simulink model "simple_dextair"  (R2018b)
settings: Solver=VariableStepAuto  StartTime=0.0  StopTime=T_simulink  RelTol=1e-3
values from neighbouring files (symbols this model uses):
  a = 1.7*10^(-6)    (= 1.7e-06)    [MAIN.m]
  delta = 0.32    [MAIN.m]
  g = 9.8    [MAIN.m]
  gamma = 3    [MAIN.m]
  k = 22.5    [MAIN.m]
  L = 0.16    [MAIN.m]
  l_0 = 10    [MAIN.m]
  lamda = 12    [MAIN.m]
  m = 2.7    [MAIN.m]
  perturpationAmp = 0    [MAIN.m]
  perturpationFreq = 0    [MAIN.m]
  PID_D_phi = PID_D    (= 19)    [MAIN.m]
  PID_D_psi = PID_D    (= 19)    [MAIN.m]
  PID_D_theta = PID_D    (= 19)    [MAIN.m]
  PID_D_x = PID_D    (= 19)    [MAIN.m]
  PID_D_y = PID_D    (= 19)    [MAIN.m]
  PID_D_z = PID_D    (= 19)    [MAIN.m]
  PID_I_phi = PID_I    (= 2.12)    [MAIN.m]
  PID_I_psi = PID_I    (= 2.12)    [MAIN.m]
  PID_I_theta = PID_I    (= 2.12)    [MAIN.m]
  PID_I_x = PID_I    (= 2.12)    [MAIN.m]
  PID_I_y = PID_I    (= 2.12)    [MAIN.m]
  PID_I_z = PID_I    (= 2.12)    [MAIN.m]
  PID_P_phi = PID_P    (= 12.71)    [MAIN.m]
  PID_P_psi = PID_P    (= 12.71)    [MAIN.m]
  PID_P_theta = PID_P    (= 12.71)    [MAIN.m]
  PID_P_x = PID_P    (= 12.71)    [MAIN.m]
  PID_P_y = PID_P    (= 12.71)    [MAIN.m]
  PID_P_z = PID_P    (= 12.71)    [MAIN.m]
  SMCONTROLTRUE = 0    [MAIN.m]
  to_motor = 0    [MAIN.m]
  W = 0.866    [MAIN.m]
  w_max = 10000000000000    [MAIN.m]
  Z_0 = m*g/k+l_0    (= 11.176)    [MAIN.m]
libraries: simulink x6
settings Model: PacingRate=3  Creator=shaabang  LastModifiedBy=shaabang
settings SolverCC: ZeroCrossControl=DisableAll  ZeroCrossAlgorithm=Adaptive
settings DebuggingCC: IgnoredZcDiagnostic=none

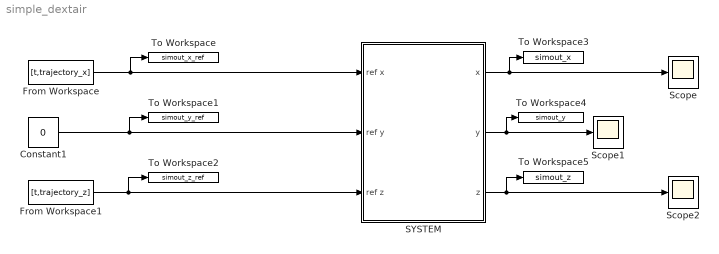
== system simple_dextair ==
  Constant1 : Constant  Value=0
  From Workspace : FromWorkspace  VariableName=[t,trajectory_x]
  From Workspace1 : FromWorkspace  VariableName=[t,trajectory_z]
  SYSTEM : Subsystem
  Scope : Scope
  Scope1 : Scope
  Scope2 : Scope
  To Workspace : ToWorkspace  VariableName=simout_x_ref  SampleTime=-1
  To Workspace1 : ToWorkspace  VariableName=simout_y_ref  SampleTime=-1
  To Workspace2 : ToWorkspace  VariableName=simout_z_ref  SampleTime=-1
  To Workspace3 : ToWorkspace  VariableName=simout_x  SampleTime=-1
  To Workspace4 : ToWorkspace  VariableName=simout_y  SampleTime=-1
  To Workspace5 : ToWorkspace  VariableName=simout_z  SampleTime=-1
  wires:
  SYSTEM/3(z) -> To Workspace5/1, Scope2/1
  SYSTEM/2(y) -> To Workspace4/1, Scope1/1
  SYSTEM/1(x) -> Scope/1, To Workspace3/1
  From Workspace1/1 -> SYSTEM/3(ref z), To Workspace2/1
  From Workspace/1 -> SYSTEM/1(ref x), To Workspace/1
  Constant1/1 -> To Workspace1/1, SYSTEM/2(ref y)

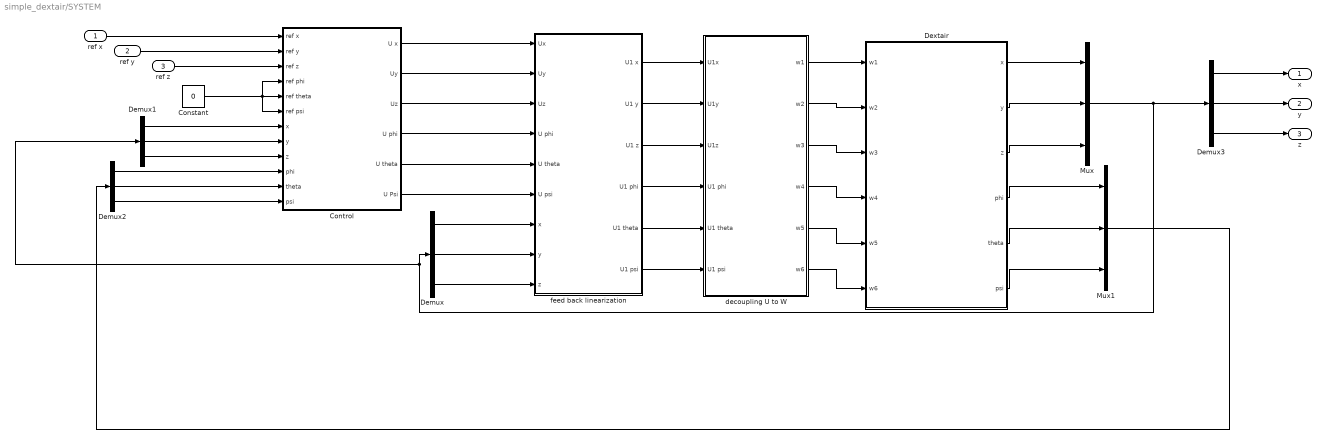
== system simple_dextair/SYSTEM ==
  ref x : Inport
  ref y : Inport  Port=2
  ref z : Inport  Port=3
  Constant : Constant  Value=0
  Control : Subsystem
  Demux{,1..3} (4 alike) : Demux  Outputs=3
  Dextair : Subsystem
  Mux : Mux  Inputs=3
  Mux1 : Mux  Inputs=3
  decoupling U to W : Subsystem
  feed back linearization : Subsystem
  x : Outport
  y : Outport  Port=2
  z : Outport  Port=3
  wires:
  decoupling U to W/5(w5) -> Dextair/5(w5)
  Demux1/2 -> Control/8(y)
  feed back linearization/2(U1 y) -> decoupling U to W/2(U1y)
  ref y/1 -> Control/2(ref y)
  Control/2(Uy) -> feed back linearization/2(Uy)
  feed back linearization/5(U1 theta) -> decoupling U to W/5(U1 theta)
  decoupling U to W/2(w2) -> Dextair/2(w2)
  decoupling U to W/4(w4) -> Dextair/4(w4)
  Dextair/5(theta) -> Mux1/2
  Control/6(U Psi) -> feed back linearization/6(U psi)
  Dextair/1(x) -> Mux/1
  Control/5(U theta) -> feed back linearization/5(U theta)
  Demux2/2 -> Control/11(theta)
  Mux/1 -> Demux3/1, Demux1/1, Demux/1
  decoupling U to W/6(w6) -> Dextair/6(w6)
  feed back linearization/3(U1 z) -> decoupling U to W/3(U1z)
  Demux1/1 -> Control/7(x)
  Demux2/3 -> Control/12(psi)
  decoupling U to W/1(w1) -> Dextair/1(w1)
  Demux/1 -> feed back linearization/7(x)
  Control/4(U phi) -> feed back linearization/4(U phi)
  Control/3(Uz) -> feed back linearization/3(Uz)
  Constant/1 -> Control/6(ref psi), Control/4(ref phi), Control/5(ref theta)
  Demux2/1 -> Control/10(phi)
  Dextair/4(phi) -> Mux1/1
  Demux1/3 -> Control/9(z)
  Dextair/6(psi) -> Mux1/3
  Control/1(U x) -> feed back linearization/1(Ux)
  feed back linearization/6(U1 psi) -> decoupling U to W/6(U1 psi)
  ref x/1 -> Control/1(ref x)
  Dextair/3(z) -> Mux/3
  ref z/1 -> Control/3(ref z)
  Demux3/2 -> y/1
  Demux/2 -> feed back linearization/8(y)
  Demux3/3 -> z/1
  Demux3/1 -> x/1
  Dextair/2(y) -> Mux/2
  feed back linearization/1(U1 x) -> decoupling U to W/1(U1x)
  feed back linearization/4(U1 phi) -> decoupling U to W/4(U1 phi)
  Demux/3 -> feed back linearization/9(z)
  decoupling U to W/3(w3) -> Dextair/3(w3)
  Mux1/1 -> Demux2/1

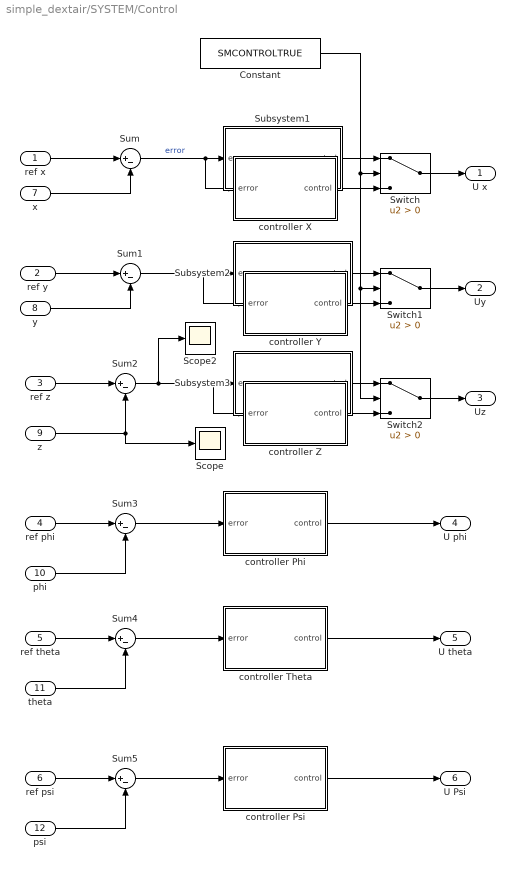
== system simple_dextair/SYSTEM/Control ==
  ref x : Inport
  ref y : Inport  Port=2
  ref z : Inport  Port=3
  ref phi : Inport  Port=4
  ref theta : Inport  Port=5
  ref psi : Inport  Port=6
  x : Inport  Port=7
  y : Inport  Port=8
  z : Inport  Port=9
  phi : Inport  Port=10
  theta : Inport  Port=11
  psi : Inport  Port=12
  Constant : Constant  Value=SMCONTROLTRUE  VectorParams1D=off
  Scope : Scope
  Scope2 : Scope
  Subsystem1 : Subsystem
  Subsystem2 : Subsystem
  Subsystem3 : Subsystem
  Sum{,1..5} (6 alike) : Sum  Inputs=|+-
  Switch : Switch  Criteria=u2 > Threshold
  Switch1 : Switch  Criteria=u2 > Threshold
  Switch2 : Switch  Criteria=u2 > Threshold
  controller Phi : Subsystem
  controller Psi : Subsystem
  controller Theta : Subsystem
  controller X : Subsystem
  controller Y : Subsystem
  controller Z : Subsystem
  U x : Outport
  Uy : Outport  Port=2
  Uz : Outport  Port=3
  U phi : Outport  Port=4
  U theta : Outport  Port=5
  U Psi : Outport  Port=6
  wires:
  controller Psi/1("control ") -> U Psi/1
  controller Theta/1("control ") -> U theta/1
  ref theta/1 -> Sum4/1
  ref y/1 -> Sum1/1
  psi/1 -> Sum5/2
  Sum2/1 -> controller Z/1("error "), Subsystem3/1(error), Scope2/1
  Sum4/1 -> controller Theta/1("error ")
  Sum5/1 -> controller Psi/1("error ")
  Sum1/1 -> controller Y/1("error "), Subsystem2/1(error)
  Sum3/1 -> controller Phi/1("error ")
  x/1 -> Sum/2
  Constant/1 -> Switch2/2, Switch1/2, Switch/2
  Switch2/1 -> Uz/1
  Subsystem1/1(control) -> Switch/1
  theta/1 -> Sum4/2
  Subsystem3/1(control) -> Switch2/1
  ref z/1 -> Sum2/1
  Switch1/1 -> Uy/1
  y/1 -> Sum1/2
  controller Phi/1("control ") -> U phi/1
  ref psi/1 -> Sum5/1
  controller X/1("control ") -> Switch/3
  z/1 -> Scope/1, Sum2/2
  Switch/1 -> U x/1
  phi/1 -> Sum3/2
  Subsystem2/1(control) -> Switch1/1
  ref phi/1 -> Sum3/1
  ref x/1 -> Sum/1
  controller Y/1("control ") -> Switch1/3
  Sum/1 -> controller X/1("error "), Subsystem1/1(error)  "error"
  controller Z/1("control ") -> Switch2/3

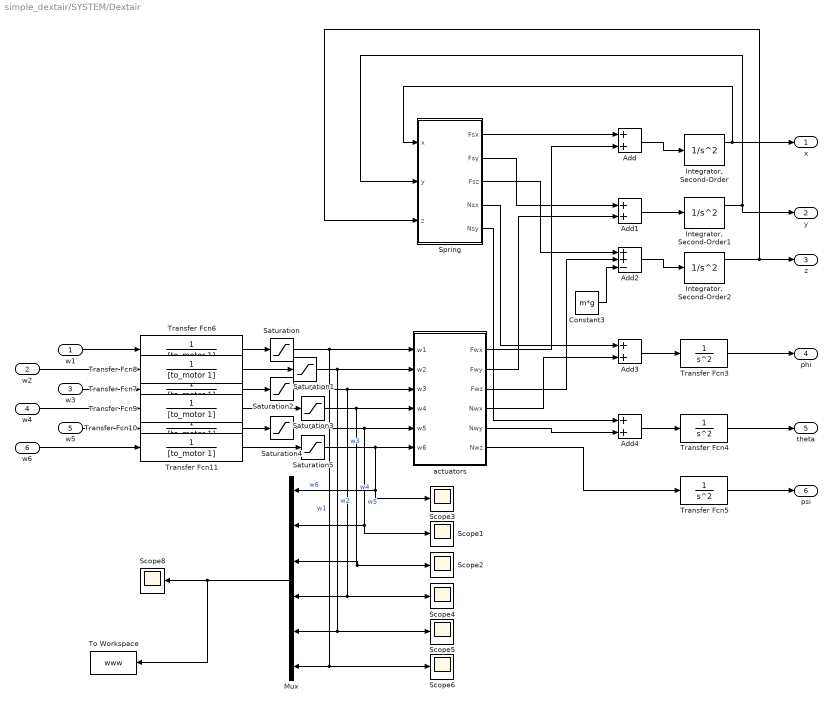
== system simple_dextair/SYSTEM/Dextair ==
  w1 : Inport
  w2 : Inport  Port=2
  w3 : Inport  Port=3
  w4 : Inport  Port=4
  w5 : Inport  Port=5
  w6 : Inport  Port=6
  Add{,1,3..4} (4 alike) : Sum
  Add2 : Sum  Inputs=++-
  Constant3 : Constant  Value=m*g
  "Integrator, Second-Order" : SecondOrderIntegrator  ICX=x0
  "Integrator, Second-Order1" : SecondOrderIntegrator  ICX=y0
  "Integrator, Second-Order2" : SecondOrderIntegrator  ICX=z0
  Mux : Mux  Inputs=6
  Saturation{,1..5} (6 alike) : Saturate  UpperLimit=w_max  LowerLimit=-w_max
  Scope{1..6,8} (7 alike) : Scope
  Spring : Subsystem
  To Workspace : ToWorkspace  VariableName=www  SampleTime=-1
  Transfer Fcn{6..11} (6 alike) : TransferFcn  Denominator=[to_motor 1]
  Transfer Fcn3 : TransferFcn  Denominator=[1 0 0]
  Transfer Fcn4 : TransferFcn  Denominator=[1 0 0]
  Transfer Fcn5 : TransferFcn  Denominator=[1 0 0]
  actuators : Subsystem
  x : Outport
  y : Outport  Port=2
  z : Outport  Port=3
  phi : Outport  Port=4
  theta : Outport  Port=5
  psi : Outport  Port=6
  wires:
  actuators/3(Fwz) -> Add2/2
  Spring/1(Fsx) -> Add/1
  Spring/5(Nsy) -> Add4/1
  Constant3/1 -> Add2/3
  Add3/1 -> Transfer Fcn3/1
  actuators/6(Nwz) -> Transfer Fcn5/1
  Add2/1 -> "Integrator, Second-Order2"/1
  Transfer Fcn5/1 -> psi/1
  Transfer Fcn3/1 -> phi/1
  Transfer Fcn4/1 -> theta/1
  "Integrator, Second-Order1"/1 -> y/1, Spring/2(y)
  Spring/2(Fsy) -> Add1/1
  actuators/1(Fwx) -> Add/2
  "Integrator, Second-Order"/1 -> x/1, Spring/1(x)
  Spring/4(Nsx) -> Add3/1
  Add1/1 -> "Integrator, Second-Order1"/1
  actuators/2(Fwy) -> Add1/2
  Spring/3(Fsz) -> Add2/1
  Add4/1 -> Transfer Fcn4/1
  Add/1 -> "Integrator, Second-Order"/1
  "Integrator, Second-Order2"/1 -> z/1, Spring/3(z)
  actuators/4(Nwx) -> Add3/2
  actuators/5(Nwy) -> Add4/2
  Transfer Fcn9/1 -> Saturation3/1
  Saturation4/1 -> actuators/5(w5), Scope1/1, Mux/2  "w5"
  Transfer Fcn7/1 -> Saturation2/1
  Saturation5/1 -> Scope3/1, Mux/1, actuators/6(w6)  "w6"
  Saturation3/1 -> actuators/4(w4), Scope2/1, Mux/3  "w4"
  Mux/1 -> To Workspace/1, Scope8/1
  Saturation/1 -> actuators/1(w1), Scope6/1, Mux/6  "w1"
  Transfer Fcn10/1 -> Saturation4/1
  Saturation2/1 -> actuators/3(w3), Scope4/1, Mux/4  "w3"
  Saturation1/1 -> actuators/2(w2), Scope5/1, Mux/5  "w2"
  Transfer Fcn8/1 -> Saturation1/1
  Transfer Fcn6/1 -> Saturation/1
  Transfer Fcn11/1 -> Saturation5/1
  w1/1 -> Transfer Fcn6/1
  w2/1 -> Transfer Fcn8/1
  w3/1 -> Transfer Fcn7/1
  w4/1 -> Transfer Fcn9/1
  w5/1 -> Transfer Fcn10/1
  w6/1 -> Transfer Fcn11/1

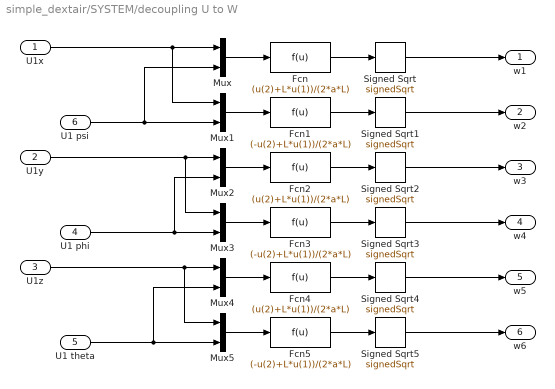
== system simple_dextair/SYSTEM/decoupling U to W ==
  U1x : Inport
  U1y : Inport  Port=2
  U1z : Inport  Port=3
  U1 phi : Inport  Port=4
  U1 theta : Inport  Port=5
  U1 psi : Inport  Port=6
  Fcn : Fcn  Expr=(u(2)+L*u(1))/(2*a*L)
  Fcn1 : Fcn  Expr=(-u(2)+L*u(1))/(2*a*L)
  Fcn2 : Fcn  Expr=(u(2)+L*u(1))/(2*a*L)
  Fcn3 : Fcn  Expr=(-u(2)+L*u(1))/(2*a*L)
  Fcn4 : Fcn  Expr=(u(2)+L*u(1))/(2*a*L)
  Fcn5 : Fcn  Expr=(-u(2)+L*u(1))/(2*a*L)
  Mux{,1..5} (6 alike) : Mux  Inputs=2
  Signed Sqrt{,1..5} (6 alike) : Sqrt  Operator=signedSqrt  SaturateOnIntegerOverflow=on
  w1 : Outport
  w2 : Outport  Port=2
  w3 : Outport  Port=3
  w4 : Outport  Port=4
  w5 : Outport  Port=5
  w6 : Outport  Port=6
  wires:
  Mux2/1 -> Fcn2/1
  Mux1/1 -> Fcn1/1
  Fcn5/1 -> Signed Sqrt5/1
  U1z/1 -> Mux5/1, Mux4/1
  Fcn3/1 -> Signed Sqrt3/1
  U1 theta/1 -> Mux4/2, Mux5/2
  Signed Sqrt2/1 -> w3/1
  Fcn/1 -> Signed Sqrt/1
  Mux3/1 -> Fcn3/1
  U1 psi/1 -> Mux/2, Mux1/2
  Fcn2/1 -> Signed Sqrt2/1
  Signed Sqrt4/1 -> w5/1
  Signed Sqrt5/1 -> w6/1
  Fcn1/1 -> Signed Sqrt1/1
  Signed Sqrt3/1 -> w4/1
  Signed Sqrt1/1 -> w2/1
  Mux/1 -> Fcn/1
  U1 phi/1 -> Mux2/2, Mux3/2
  U1x/1 -> Mux1/1, Mux/1
  U1y/1 -> Mux3/1, Mux2/1
  Mux5/1 -> Fcn5/1
  Fcn4/1 -> Signed Sqrt4/1
  Signed Sqrt/1 -> w1/1
  Mux4/1 -> Fcn4/1

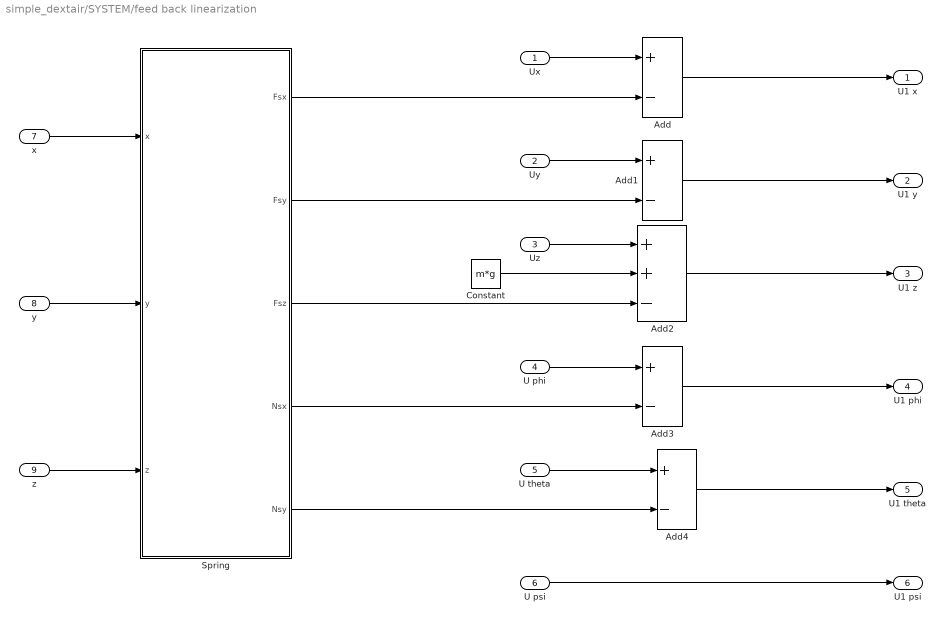
== system simple_dextair/SYSTEM/feed back linearization ==
  Ux : Inport
  Uy : Inport  Port=2
  Uz : Inport  Port=3
  U phi : Inport  Port=4
  U theta : Inport  Port=5
  U psi : Inport  Port=6
  x : Inport  Port=7
  y : Inport  Port=8
  z : Inport  Port=9
  Add{,1,3..4} (4 alike) : Sum  Inputs=+-
  Add2 : Sum  Inputs=++-
  Constant : Constant  Value=m*g
  Spring : Subsystem
  U1 x : Outport
  U1 y : Outport  Port=2
  U1 z : Outport  Port=3
  U1 phi : Outport  Port=4
  U1 theta : Outport  Port=5
  U1 psi : Outport  Port=6
  wires:
  U psi/1 -> U1 psi/1
  Add/1 -> U1 x/1
  Spring/4(Nsx) -> Add3/2
  Uy/1 -> Add1/1
  z/1 -> Spring/3(z)
  y/1 -> Spring/2(y)
  Spring/5(Nsy) -> Add4/2
  Constant/1 -> Add2/2
  U phi/1 -> Add3/1
  Add2/1 -> U1 z/1
  Add4/1 -> U1 theta/1
  Spring/1(Fsx) -> Add/2
  U theta/1 -> Add4/1
  x/1 -> Spring/1(x)
  Spring/3(Fsz) -> Add2/3
  Ux/1 -> Add/1
  Add1/1 -> U1 y/1
  Add3/1 -> U1 phi/1
  Uz/1 -> Add2/1
  Spring/2(Fsy) -> Add1/2

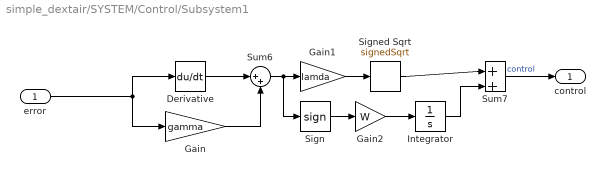
== system simple_dextair/SYSTEM/Control/Subsystem1 ==
  error : Inport
  Derivative : Derivative
  Gain : Gain  Gain=gamma
  Gain1 : Gain  Gain=lamda
  Gain2 : Gain  Gain=W
  Integrator : Integrator
  Sign : Signum
  Signed Sqrt : Sqrt  Operator=signedSqrt  SaturateOnIntegerOverflow=on
  Sum6 : Sum  Inputs=|++
  Sum7 : Sum  Inputs=|++
  control : Outport
  wires:
  Sum7/1 -> control/1  "control"
  Sign/1 -> Gain2/1
  error/1 -> Derivative/1, Gain/1
  Derivative/1 -> Sum6/1
  Gain2/1 -> Integrator/1
  Signed Sqrt/1 -> Sum7/1
  Gain/1 -> Sum6/2
  Gain1/1 -> Signed Sqrt/1
  Sum6/1 -> Gain1/1, Sign/1
  Integrator/1 -> Sum7/2

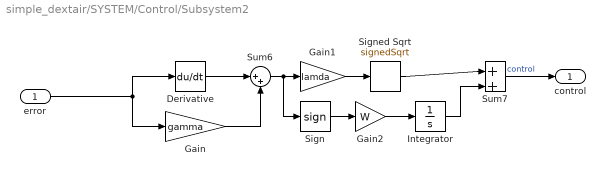
== system simple_dextair/SYSTEM/Control/Subsystem2 ==
  error : Inport
  Derivative : Derivative
  Gain : Gain  Gain=gamma
  Gain1 : Gain  Gain=lamda
  Gain2 : Gain  Gain=W
  Integrator : Integrator
  Sign : Signum
  Signed Sqrt : Sqrt  Operator=signedSqrt  SaturateOnIntegerOverflow=on
  Sum6 : Sum  Inputs=|++
  Sum7 : Sum  Inputs=|++
  control : Outport
  wires:
  Integrator/1 -> Sum7/2
  Sum6/1 -> Sign/1, Gain1/1
  Gain1/1 -> Signed Sqrt/1
  Gain/1 -> Sum6/2
  Signed Sqrt/1 -> Sum7/1
  Gain2/1 -> Integrator/1
  Derivative/1 -> Sum6/1
  error/1 -> Gain/1, Derivative/1
  Sign/1 -> Gain2/1
  Sum7/1 -> control/1  "control"

== system simple_dextair/SYSTEM/Control/Subsystem3 ==
  error : Inport
  Derivative : Derivative
  Gain : Gain  Gain=gamma
  Gain1 : Gain  Gain=lamda
  Gain2 : Gain  Gain=W
  Integrator : Integrator
  Sign : Signum
  Signed Sqrt : Sqrt  Operator=signedSqrt  SaturateOnIntegerOverflow=on
  Sum6 : Sum  Inputs=|++
  Sum7 : Sum  Inputs=|++
  control : Outport
  wires:
  Sum7/1 -> control/1  "control"
  Sign/1 -> Gain2/1
  error/1 -> Derivative/1, Gain/1
  Derivative/1 -> Sum6/1
  Gain2/1 -> Integrator/1
  Signed Sqrt/1 -> Sum7/1
  Gain/1 -> Sum6/2
  Gain1/1 -> Signed Sqrt/1
  Sum6/1 -> Gain1/1, Sign/1
  Integrator/1 -> Sum7/2

== system simple_dextair/SYSTEM/Control/controller Phi ==
  "error " : Inport
  PID Controller : simulink/Continuous/PID Controller  Controller=PID  Form=Parallel  TimeDomain=Continuous-time  SampleTime=-1  IntegratorMethod=Forward Euler  FilterMethod=Forward Euler  ControllerParametersSource=internal  P=PID_P_phi  I=PID_I_phi  D=PID_D_phi  UseFilter=on  N=100  TunerSelectOption=Transfer Function Based (PID Tuner App)  InitialConditionSource=internal  InitialConditionForIntegrator=0  InitialConditionForFilter=0  DifferentiatorICPrevScaledInput=0  ExternalReset=none  TrackingMode=off  Kt=1  LimitOutput=off  UpperSaturationLimit=inf  LowerSaturationLimit=-inf  LinearizeAsGain=on  AntiWindupMode=none  Kb=1  POutMin=[]  POutMax=[]  IOutMin=[]  IOutMax=[]  DOutMin=[]  DOutMax=[]  NOutMin=[]  NOutMax=[]  SumOutMin=[]  SumOutMax=[]  SaturationOutMin=[]  SaturationOutMax=[]  PParamMin=[]  PParamMax=[]  IParamMin=[]  IParamMax=[]  DParamMin=[]  DParamMax=[]  NParamMin=[]  NParamMax=[]  KbParamMin=[]  KbParamMax=[]  KtParamMin=[]  KtParamMax=[]  KbOutMin=[]  KbOutMax=[]  KtOutMin=[]  KtOutMax=[]  IntegratorOutMin=[]  IntegratorOutMax=[]  FilterOutMin=[]  FilterOutMax=[]  SumI1OutMin=[]  SumI1OutMax=[]  SumI2OutMin=[]  SumI2OutMax=[]  SumI3OutMin=[]  SumI3OutMax=[]  SumI4OutMin=[]  SumI4OutMax=[]  SumDOutMin=[]  SumDOutMax=[]  DifferentiatorOutMin=[]  DifferentiatorOutMax=[]  FilterDiffOutCoefMin=[]  FilterDiffOutCoefMax=[]  ReciprocalOutMin=[]  ReciprocalOutMax=[]  SumDenOutMin=[]  SumDenOutMax=[]  SumNumOutMin=[]  SumNumOutMax=[]  DivideOutMin=[]  DivideOutMax=[]  IntegratorContinuousStateAttributes=''  IntegratorStateMustResolveToSignalObject=off  IntegratorRTWStateStorageClass=Auto  FilterContinuousStateAttributes=''  FilterStateMustResolveToSignalObject=off  FilterRTWStateStorageClass=Auto  ParallelPVariant=InternalParameters  IdealPVariant=Disabled  IVariant=InternalParameters  DVariant=InternalParameters  IntegratorVariant=Continuous  SatVariant=Disabled  AWVariant=Passthrough  PCopyVariant=Disabled  TRVariant=Disabled  FdbkBlocksVariant=Forward  IdealPFdbkVariant=Disabled  SatFdbkVariant=Disabled  DerivativeFilterVariant=ContFilter  NVariant=InternalParameters  NCopyVariant=Disabled  FilterICVariant=InternalICsFilter  IntegratorICVariant=InternalICs  ExternalResetVariant=Disabled  TRSumVariant=Passthrough  SumFdbkVariant=Disabled  SumVariant=Sum_PID
  "control " : Outport
  wires:
  PID Controller/1 -> "control "/1
  "error "/1 -> PID Controller/1

== system simple_dextair/SYSTEM/Control/controller Psi ==
  "error " : Inport
  PID Controller : simulink/Continuous/PID Controller  Controller=PID  Form=Parallel  TimeDomain=Continuous-time  SampleTime=-1  IntegratorMethod=Forward Euler  FilterMethod=Forward Euler  ControllerParametersSource=internal  P=PID_P_psi  I=PID_I_psi  D=PID_D_psi  UseFilter=on  N=100  TunerSelectOption=Transfer Function Based (PID Tuner App)  InitialConditionSource=internal  InitialConditionForIntegrator=0  InitialConditionForFilter=0  DifferentiatorICPrevScaledInput=0  ExternalReset=none  TrackingMode=off  Kt=1  LimitOutput=off  UpperSaturationLimit=inf  LowerSaturationLimit=-inf  LinearizeAsGain=on  AntiWindupMode=none  Kb=1  POutMin=[]  POutMax=[]  IOutMin=[]  IOutMax=[]  DOutMin=[]  DOutMax=[]  NOutMin=[]  NOutMax=[]  SumOutMin=[]  SumOutMax=[]  SaturationOutMin=[]  SaturationOutMax=[]  PParamMin=[]  PParamMax=[]  IParamMin=[]  IParamMax=[]  DParamMin=[]  DParamMax=[]  NParamMin=[]  NParamMax=[]  KbParamMin=[]  KbParamMax=[]  KtParamMin=[]  KtParamMax=[]  KbOutMin=[]  KbOutMax=[]  KtOutMin=[]  KtOutMax=[]  IntegratorOutMin=[]  IntegratorOutMax=[]  FilterOutMin=[]  FilterOutMax=[]  SumI1OutMin=[]  SumI1OutMax=[]  SumI2OutMin=[]  SumI2OutMax=[]  SumI3OutMin=[]  SumI3OutMax=[]  SumI4OutMin=[]  SumI4OutMax=[]  SumDOutMin=[]  SumDOutMax=[]  DifferentiatorOutMin=[]  DifferentiatorOutMax=[]  FilterDiffOutCoefMin=[]  FilterDiffOutCoefMax=[]  ReciprocalOutMin=[]  ReciprocalOutMax=[]  SumDenOutMin=[]  SumDenOutMax=[]  SumNumOutMin=[]  SumNumOutMax=[]  DivideOutMin=[]  DivideOutMax=[]  IntegratorContinuousStateAttributes=''  IntegratorStateMustResolveToSignalObject=off  IntegratorRTWStateStorageClass=Auto  FilterContinuousStateAttributes=''  FilterStateMustResolveToSignalObject=off  FilterRTWStateStorageClass=Auto  ParallelPVariant=InternalParameters  IdealPVariant=Disabled  IVariant=InternalParameters  DVariant=InternalParameters  IntegratorVariant=Continuous  SatVariant=Disabled  AWVariant=Passthrough  PCopyVariant=Disabled  TRVariant=Disabled  FdbkBlocksVariant=Forward  IdealPFdbkVariant=Disabled  SatFdbkVariant=Disabled  DerivativeFilterVariant=ContFilter  NVariant=InternalParameters  NCopyVariant=Disabled  FilterICVariant=InternalICsFilter  IntegratorICVariant=InternalICs  ExternalResetVariant=Disabled  TRSumVariant=Passthrough  SumFdbkVariant=Disabled  SumVariant=Sum_PID
  "control " : Outport
  wires:
  PID Controller/1 -> "control "/1
  "error "/1 -> PID Controller/1

== system simple_dextair/SYSTEM/Control/controller Theta ==
  "error " : Inport
  PID Controller : simulink/Continuous/PID Controller  Controller=PID  Form=Parallel  TimeDomain=Continuous-time  SampleTime=-1  IntegratorMethod=Forward Euler  FilterMethod=Forward Euler  ControllerParametersSource=internal  P=PID_P_theta  I=PID_I_theta  D=PID_D_theta  UseFilter=on  N=100  TunerSelectOption=Transfer Function Based (PID Tuner App)  InitialConditionSource=internal  InitialConditionForIntegrator=0  InitialConditionForFilter=0  DifferentiatorICPrevScaledInput=0  ExternalReset=none  TrackingMode=off  Kt=1  LimitOutput=off  UpperSaturationLimit=inf  LowerSaturationLimit=-inf  LinearizeAsGain=on  AntiWindupMode=none  Kb=1  POutMin=[]  POutMax=[]  IOutMin=[]  IOutMax=[]  DOutMin=[]  DOutMax=[]  NOutMin=[]  NOutMax=[]  SumOutMin=[]  SumOutMax=[]  SaturationOutMin=[]  SaturationOutMax=[]  PParamMin=[]  PParamMax=[]  IParamMin=[]  IParamMax=[]  DParamMin=[]  DParamMax=[]  NParamMin=[]  NParamMax=[]  KbParamMin=[]  KbParamMax=[]  KtParamMin=[]  KtParamMax=[]  KbOutMin=[]  KbOutMax=[]  KtOutMin=[]  KtOutMax=[]  IntegratorOutMin=[]  IntegratorOutMax=[]  FilterOutMin=[]  FilterOutMax=[]  SumI1OutMin=[]  SumI1OutMax=[]  SumI2OutMin=[]  SumI2OutMax=[]  SumI3OutMin=[]  SumI3OutMax=[]  SumI4OutMin=[]  SumI4OutMax=[]  SumDOutMin=[]  SumDOutMax=[]  DifferentiatorOutMin=[]  DifferentiatorOutMax=[]  FilterDiffOutCoefMin=[]  FilterDiffOutCoefMax=[]  ReciprocalOutMin=[]  ReciprocalOutMax=[]  SumDenOutMin=[]  SumDenOutMax=[]  SumNumOutMin=[]  SumNumOutMax=[]  DivideOutMin=[]  DivideOutMax=[]  IntegratorContinuousStateAttributes=''  IntegratorStateMustResolveToSignalObject=off  IntegratorRTWStateStorageClass=Auto  FilterContinuousStateAttributes=''  FilterStateMustResolveToSignalObject=off  FilterRTWStateStorageClass=Auto  ParallelPVariant=InternalParameters  IdealPVariant=Disabled  IVariant=InternalParameters  DVariant=InternalParameters  IntegratorVariant=Continuous  SatVariant=Disabled  AWVariant=Passthrough  PCopyVariant=Disabled  TRVariant=Disabled  FdbkBlocksVariant=Forward  IdealPFdbkVariant=Disabled  SatFdbkVariant=Disabled  DerivativeFilterVariant=ContFilter  NVariant=InternalParameters  NCopyVariant=Disabled  FilterICVariant=InternalICsFilter  IntegratorICVariant=InternalICs  ExternalResetVariant=Disabled  TRSumVariant=Passthrough  SumFdbkVariant=Disabled  SumVariant=Sum_PID
  "control " : Outport
  wires:
  PID Controller/1 -> "control "/1
  "error "/1 -> PID Controller/1

== system simple_dextair/SYSTEM/Control/controller X ==
  "error " : Inport
  PID Controller : simulink/Continuous/PID Controller  Controller=PID  Form=Parallel  TimeDomain=Continuous-time  SampleTime=-1  IntegratorMethod=Forward Euler  FilterMethod=Forward Euler  ControllerParametersSource=internal  P=PID_P_x  I=PID_I_x  D=PID_D_x  UseFilter=on  N=100  TunerSelectOption=Transfer Function Based (PID Tuner App)  InitialConditionSource=internal  InitialConditionForIntegrator=0  InitialConditionForFilter=0  DifferentiatorICPrevScaledInput=0  ExternalReset=none  TrackingMode=off  Kt=1  LimitOutput=off  UpperSaturationLimit=inf  LowerSaturationLimit=-inf  LinearizeAsGain=on  AntiWindupMode=none  Kb=1  POutMin=[]  POutMax=[]  IOutMin=[]  IOutMax=[]  DOutMin=[]  DOutMax=[]  NOutMin=[]  NOutMax=[]  SumOutMin=[]  SumOutMax=[]  SaturationOutMin=[]  SaturationOutMax=[]  PParamMin=[]  PParamMax=[]  IParamMin=[]  IParamMax=[]  DParamMin=[]  DParamMax=[]  NParamMin=[]  NParamMax=[]  KbParamMin=[]  KbParamMax=[]  KtParamMin=[]  KtParamMax=[]  KbOutMin=[]  KbOutMax=[]  KtOutMin=[]  KtOutMax=[]  IntegratorOutMin=[]  IntegratorOutMax=[]  FilterOutMin=[]  FilterOutMax=[]  SumI1OutMin=[]  SumI1OutMax=[]  SumI2OutMin=[]  SumI2OutMax=[]  SumI3OutMin=[]  SumI3OutMax=[]  SumI4OutMin=[]  SumI4OutMax=[]  SumDOutMin=[]  SumDOutMax=[]  DifferentiatorOutMin=[]  DifferentiatorOutMax=[]  FilterDiffOutCoefMin=[]  FilterDiffOutCoefMax=[]  ReciprocalOutMin=[]  ReciprocalOutMax=[]  SumDenOutMin=[]  SumDenOutMax=[]  SumNumOutMin=[]  SumNumOutMax=[]  DivideOutMin=[]  DivideOutMax=[]  IntegratorContinuousStateAttributes=''  IntegratorStateMustResolveToSignalObject=off  IntegratorRTWStateStorageClass=Auto  FilterContinuousStateAttributes=''  FilterStateMustResolveToSignalObject=off  FilterRTWStateStorageClass=Auto  ParallelPVariant=InternalParameters  IdealPVariant=Disabled  IVariant=InternalParameters  DVariant=InternalParameters  IntegratorVariant=Continuous  SatVariant=Disabled  AWVariant=Passthrough  PCopyVariant=Disabled  TRVariant=Disabled  FdbkBlocksVariant=Forward  IdealPFdbkVariant=Disabled  SatFdbkVariant=Disabled  DerivativeFilterVariant=ContFilter  NVariant=InternalParameters  NCopyVariant=Disabled  FilterICVariant=InternalICsFilter  IntegratorICVariant=InternalICs  ExternalResetVariant=Disabled  TRSumVariant=Passthrough  SumFdbkVariant=Disabled  SumVariant=Sum_PID
  "control " : Outport
  wires:
  PID Controller/1 -> "control "/1
  "error "/1 -> PID Controller/1

== system simple_dextair/SYSTEM/Control/controller Y ==
  "error " : Inport
  PID Controller : simulink/Continuous/PID Controller  Controller=PID  Form=Parallel  TimeDomain=Continuous-time  SampleTime=-1  IntegratorMethod=Forward Euler  FilterMethod=Forward Euler  ControllerParametersSource=internal  P=PID_P_y  I=PID_I_y  D=PID_D_y  UseFilter=on  N=100  TunerSelectOption=Transfer Function Based (PID Tuner App)  InitialConditionSource=internal  InitialConditionForIntegrator=0  InitialConditionForFilter=0  DifferentiatorICPrevScaledInput=0  ExternalReset=none  TrackingMode=off  Kt=1  LimitOutput=off  UpperSaturationLimit=inf  LowerSaturationLimit=-inf  LinearizeAsGain=on  AntiWindupMode=none  Kb=1  POutMin=[]  POutMax=[]  IOutMin=[]  IOutMax=[]  DOutMin=[]  DOutMax=[]  NOutMin=[]  NOutMax=[]  SumOutMin=[]  SumOutMax=[]  SaturationOutMin=[]  SaturationOutMax=[]  PParamMin=[]  PParamMax=[]  IParamMin=[]  IParamMax=[]  DParamMin=[]  DParamMax=[]  NParamMin=[]  NParamMax=[]  KbParamMin=[]  KbParamMax=[]  KtParamMin=[]  KtParamMax=[]  KbOutMin=[]  KbOutMax=[]  KtOutMin=[]  KtOutMax=[]  IntegratorOutMin=[]  IntegratorOutMax=[]  FilterOutMin=[]  FilterOutMax=[]  SumI1OutMin=[]  SumI1OutMax=[]  SumI2OutMin=[]  SumI2OutMax=[]  SumI3OutMin=[]  SumI3OutMax=[]  SumI4OutMin=[]  SumI4OutMax=[]  SumDOutMin=[]  SumDOutMax=[]  DifferentiatorOutMin=[]  DifferentiatorOutMax=[]  FilterDiffOutCoefMin=[]  FilterDiffOutCoefMax=[]  ReciprocalOutMin=[]  ReciprocalOutMax=[]  SumDenOutMin=[]  SumDenOutMax=[]  SumNumOutMin=[]  SumNumOutMax=[]  DivideOutMin=[]  DivideOutMax=[]  IntegratorContinuousStateAttributes=''  IntegratorStateMustResolveToSignalObject=off  IntegratorRTWStateStorageClass=Auto  FilterContinuousStateAttributes=''  FilterStateMustResolveToSignalObject=off  FilterRTWStateStorageClass=Auto  ParallelPVariant=InternalParameters  IdealPVariant=Disabled  IVariant=InternalParameters  DVariant=InternalParameters  IntegratorVariant=Continuous  SatVariant=Disabled  AWVariant=Passthrough  PCopyVariant=Disabled  TRVariant=Disabled  FdbkBlocksVariant=Forward  IdealPFdbkVariant=Disabled  SatFdbkVariant=Disabled  DerivativeFilterVariant=ContFilter  NVariant=InternalParameters  NCopyVariant=Disabled  FilterICVariant=InternalICsFilter  IntegratorICVariant=InternalICs  ExternalResetVariant=Disabled  TRSumVariant=Passthrough  SumFdbkVariant=Disabled  SumVariant=Sum_PID
  "control " : Outport
  wires:
  "error "/1 -> PID Controller/1
  PID Controller/1 -> "control "/1

== system simple_dextair/SYSTEM/Control/controller Z ==
  "error " : Inport
  PID Controller : simulink/Continuous/PID Controller  Controller=PID  Form=Parallel  TimeDomain=Continuous-time  SampleTime=-1  IntegratorMethod=Forward Euler  FilterMethod=Forward Euler  ControllerParametersSource=internal  P=PID_P_z  I=PID_I_z  D=PID_D_z  UseFilter=on  N=100  TunerSelectOption=Transfer Function Based (PID Tuner App)  InitialConditionSource=internal  InitialConditionForIntegrator=0  InitialConditionForFilter=0  DifferentiatorICPrevScaledInput=0  ExternalReset=none  TrackingMode=off  Kt=1  LimitOutput=off  UpperSaturationLimit=inf  LowerSaturationLimit=-inf  LinearizeAsGain=on  AntiWindupMode=none  Kb=1  POutMin=[]  POutMax=[]  IOutMin=[]  IOutMax=[]  DOutMin=[]  DOutMax=[]  NOutMin=[]  NOutMax=[]  SumOutMin=[]  SumOutMax=[]  SaturationOutMin=[]  SaturationOutMax=[]  PParamMin=[]  PParamMax=[]  IParamMin=[]  IParamMax=[]  DParamMin=[]  DParamMax=[]  NParamMin=[]  NParamMax=[]  KbParamMin=[]  KbParamMax=[]  KtParamMin=[]  KtParamMax=[]  KbOutMin=[]  KbOutMax=[]  KtOutMin=[]  KtOutMax=[]  IntegratorOutMin=[]  IntegratorOutMax=[]  FilterOutMin=[]  FilterOutMax=[]  SumI1OutMin=[]  SumI1OutMax=[]  SumI2OutMin=[]  SumI2OutMax=[]  SumI3OutMin=[]  SumI3OutMax=[]  SumI4OutMin=[]  SumI4OutMax=[]  SumDOutMin=[]  SumDOutMax=[]  DifferentiatorOutMin=[]  DifferentiatorOutMax=[]  FilterDiffOutCoefMin=[]  FilterDiffOutCoefMax=[]  ReciprocalOutMin=[]  ReciprocalOutMax=[]  SumDenOutMin=[]  SumDenOutMax=[]  SumNumOutMin=[]  SumNumOutMax=[]  DivideOutMin=[]  DivideOutMax=[]  IntegratorContinuousStateAttributes=''  IntegratorStateMustResolveToSignalObject=off  IntegratorRTWStateStorageClass=Auto  FilterContinuousStateAttributes=''  FilterStateMustResolveToSignalObject=off  FilterRTWStateStorageClass=Auto  ParallelPVariant=InternalParameters  IdealPVariant=Disabled  IVariant=InternalParameters  DVariant=InternalParameters  IntegratorVariant=Continuous  SatVariant=Disabled  AWVariant=Passthrough  PCopyVariant=Disabled  TRVariant=Disabled  FdbkBlocksVariant=Forward  IdealPFdbkVariant=Disabled  SatFdbkVariant=Disabled  DerivativeFilterVariant=ContFilter  NVariant=InternalParameters  NCopyVariant=Disabled  FilterICVariant=InternalICsFilter  IntegratorICVariant=InternalICs  ExternalResetVariant=Disabled  TRSumVariant=Passthrough  SumFdbkVariant=Disabled  SumVariant=Sum_PID
  "control " : Outport
  wires:
  PID Controller/1 -> "control "/1
  "error "/1 -> PID Controller/1

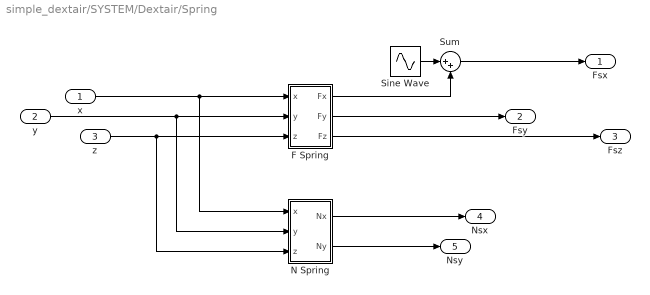
== system simple_dextair/SYSTEM/Dextair/Spring ==
  x : Inport
  y : Inport  Port=2
  z : Inport  Port=3
  F Spring : Subsystem
  N Spring : Subsystem
  Sine Wave : Sin  Amplitude=perturpationAmp  Frequency=perturpationFreq  SampleTime=0
  Sum : Sum  Inputs=|++
  Fsx : Outport
  Fsy : Outport  Port=2
  Fsz : Outport  Port=3
  Nsx : Outport  Port=4
  Nsy : Outport  Port=5
  wires:
  x/1 -> N Spring/1(x), F Spring/1(x)
  N Spring/2(Ny) -> Nsy/1
  F Spring/2(Fy) -> Fsy/1
  N Spring/1("Nx ") -> Nsx/1
  F Spring/3(Fz) -> Fsz/1
  y/1 -> N Spring/2(y), F Spring/2(y)
  z/1 -> N Spring/3(z), F Spring/3(z)
  Sine Wave/1 -> Sum/1
  F Spring/1(Fx) -> Sum/2
  Sum/1 -> Fsx/1

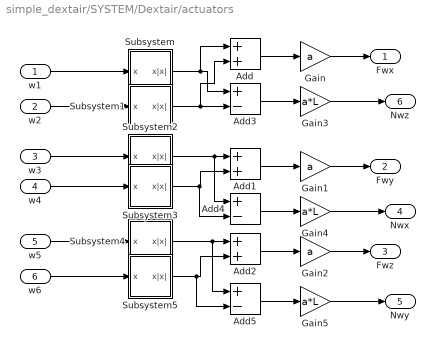
== system simple_dextair/SYSTEM/Dextair/actuators ==
  w1 : Inport
  w2 : Inport  Port=2
  w3 : Inport  Port=3
  w4 : Inport  Port=4
  w5 : Inport  Port=5
  w6 : Inport  Port=6
  Add : Sum
  Add1 : Sum
  Add2 : Sum
  Add3 : Sum  Inputs=+-
  Add4 : Sum  Inputs=+-
  Add5 : Sum  Inputs=+-
  Gain : Gain  Gain=a
  Gain1 : Gain  Gain=a
  Gain2 : Gain  Gain=a
  Gain3 : Gain  Gain=a*L
  Gain4 : Gain  Gain=a*L
  Gain5 : Gain  Gain=a*L
  Subsystem : Subsystem
  Subsystem1 : Subsystem
  Subsystem2 : Subsystem
  Subsystem3 : Subsystem
  Subsystem4 : Subsystem
  Subsystem5 : Subsystem
  Fwx : Outport
  Fwy : Outport  Port=2
  Fwz : Outport  Port=3
  Nwx : Outport  Port=4
  Nwy : Outport  Port=5
  Nwz : Outport  Port=6
  wires:
  Subsystem4/1(x|x|) -> Add5/1, Add2/1
  Gain1/1 -> Fwy/1
  Subsystem2/1(x|x|) -> Add4/1, Add1/1
  Gain5/1 -> Nwy/1
  w5/1 -> Subsystem4/1(x)
  Add5/1 -> Gain5/1
  Gain4/1 -> Nwx/1
  Add2/1 -> Gain2/1
  w3/1 -> Subsystem2/1(x)
  Add/1 -> Gain/1
  Add4/1 -> Gain4/1
  Gain2/1 -> Fwz/1
  Subsystem3/1(x|x|) -> Add4/2, Add1/2
  Gain3/1 -> Nwz/1
  Subsystem1/1(x|x|) -> Add3/2, Add/2
  Add1/1 -> Gain1/1
  Subsystem/1(x|x|) -> Add3/1, Add/1
  w2/1 -> Subsystem1/1(x)
  Add3/1 -> Gain3/1
  w1/1 -> Subsystem/1(x)
  Gain/1 -> Fwx/1
  Subsystem5/1(x|x|) -> Add5/2, Add2/2
  w4/1 -> Subsystem3/1(x)
  w6/1 -> Subsystem5/1(x)

== system simple_dextair/SYSTEM/feed back linearization/Spring ==
  x : Inport
  y : Inport  Port=2
  z : Inport  Port=3
  F Spring : Subsystem
  N Spring : Subsystem
  Fsx : Outport
  Fsy : Outport  Port=2
  Fsz : Outport  Port=3
  Nsx : Outport  Port=4
  Nsy : Outport  Port=5
  wires:
  x/1 -> N Spring/1(x), F Spring/1(x)
  N Spring/2(Ny) -> Nsy/1
  F Spring/2(Fy) -> Fsy/1
  N Spring/1("Nx ") -> Nsx/1
  F Spring/3(Fz) -> Fsz/1
  y/1 -> N Spring/2(y), F Spring/2(y)
  z/1 -> N Spring/3(z), F Spring/3(z)
  F Spring/1(Fx) -> Fsx/1

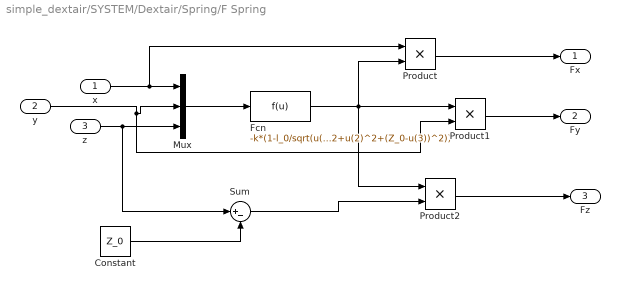
== system simple_dextair/SYSTEM/Dextair/Spring/F Spring ==
  x : Inport
  y : Inport  Port=2
  z : Inport  Port=3
  Constant : Constant  Value=Z_0
  Fcn : Fcn  Expr=-k*(1-l_0/sqrt(u(1)^2+u(2)^2+(Z_0-u(3))^2))
  Mux : Mux  Inputs=3
  Product : Product
  Product1 : Product
  Product2 : Product
  Sum : Sum  Inputs=|+-
  Fx : Outport
  Fy : Outport  Port=2
  Fz : Outport  Port=3
  wires:
  Sum/1 -> Product2/2
  Fcn/1 -> Product/2, Product2/1, Product1/1
  Mux/1 -> Fcn/1
  z/1 -> Sum/1, Mux/3
  Product/1 -> Fx/1
  Product2/1 -> Fz/1
  x/1 -> Product/1, Mux/1
  Constant/1 -> Sum/2
  Product1/1 -> Fy/1
  y/1 -> Product1/2, Mux/2

== system simple_dextair/SYSTEM/Dextair/Spring/N Spring ==
  x : Inport
  y : Inport  Port=2
  z : Inport  Port=3
  Fcn : Fcn  Expr=-k*(1-l_0/sqrt(u(1)^2+u(2)^2+(Z_0-u(3))^2))
  Gain : Gain  Gain=delta
  Gain1 : Gain  Gain=-1
  Mux : Mux  Inputs=3
  Product : Product
  Product1 : Product
  "Nx " : Outport
  Ny : Outport  Port=2
  wires:
  y/1 -> Mux/2, Product1/2
  Product1/1 -> Gain1/1
  x/1 -> Mux/1, Product/1
  Product/1 -> Ny/1
  z/1 -> Mux/3
  Mux/1 -> Fcn/1
  Fcn/1 -> Gain/1
  Gain/1 -> Product1/1, Product/2
  Gain1/1 -> "Nx "/1

== system simple_dextair/SYSTEM/Dextair/actuators/Subsystem ==
  x : Inport
  Abs : Abs
  Product : Product
  x|x| : Outport
  wires:
  Product/1 -> x|x|/1
  Abs/1 -> Product/1
  x/1 -> Abs/1, Product/2

== system simple_dextair/SYSTEM/Dextair/actuators/Subsystem1 ==
  x : Inport
  Abs : Abs
  Product : Product
  x|x| : Outport
  wires:
  x/1 -> Product/2, Abs/1
  Abs/1 -> Product/1
  Product/1 -> x|x|/1

== system simple_dextair/SYSTEM/Dextair/actuators/Subsystem2 ==
  x : Inport
  Abs : Abs
  Product : Product
  x|x| : Outport
  wires:
  Product/1 -> x|x|/1
  Abs/1 -> Product/1
  x/1 -> Abs/1, Product/2

== system simple_dextair/SYSTEM/Dextair/actuators/Subsystem3 ==
  x : Inport
  Abs : Abs
  Product : Product
  x|x| : Outport
  wires:
  x/1 -> Product/2, Abs/1
  Abs/1 -> Product/1
  Product/1 -> x|x|/1

== system simple_dextair/SYSTEM/Dextair/actuators/Subsystem4 ==
  x : Inport
  Abs : Abs
  Product : Product
  x|x| : Outport
  wires:
  Product/1 -> x|x|/1
  Abs/1 -> Product/1
  x/1 -> Abs/1, Product/2

== system simple_dextair/SYSTEM/Dextair/actuators/Subsystem5 ==
  x : Inport
  Abs : Abs
  Product : Product
  x|x| : Outport
  wires:
  x/1 -> Product/2, Abs/1
  Abs/1 -> Product/1
  Product/1 -> x|x|/1

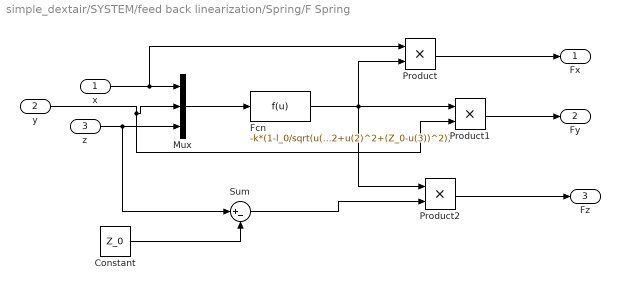
== system simple_dextair/SYSTEM/feed back linearization/Spring/F Spring ==
  x : Inport
  y : Inport  Port=2
  z : Inport  Port=3
  Constant : Constant  Value=Z_0
  Fcn : Fcn  Expr=-k*(1-l_0/sqrt(u(1)^2+u(2)^2+(Z_0-u(3))^2))
  Mux : Mux  Inputs=3
  Product : Product
  Product1 : Product
  Product2 : Product
  Sum : Sum  Inputs=|+-
  Fx : Outport
  Fy : Outport  Port=2
  Fz : Outport  Port=3
  wires:
  Sum/1 -> Product2/2
  Fcn/1 -> Product/2, Product2/1, Product1/1
  Mux/1 -> Fcn/1
  z/1 -> Sum/1, Mux/3
  Product/1 -> Fx/1
  Product2/1 -> Fz/1
  x/1 -> Product/1, Mux/1
  Constant/1 -> Sum/2
  Product1/1 -> Fy/1
  y/1 -> Product1/2, Mux/2

== system simple_dextair/SYSTEM/feed back linearization/Spring/N Spring ==
  x : Inport
  y : Inport  Port=2
  z : Inport  Port=3
  Fcn : Fcn  Expr=-k*(1-l_0/sqrt(u(1)^2+u(2)^2+(Z_0-u(3))^2))
  Gain : Gain  Gain=delta
  Gain1 : Gain  Gain=-1
  Mux : Mux  Inputs=3
  Product : Product
  Product1 : Product
  "Nx " : Outport
  Ny : Outport  Port=2
  wires:
  y/1 -> Mux/2, Product1/2
  Product1/1 -> Gain1/1
  x/1 -> Mux/1, Product/1
  Product/1 -> Ny/1
  z/1 -> Mux/3
  Mux/1 -> Fcn/1
  Fcn/1 -> Gain/1
  Gain/1 -> Product1/1, Product/2
  Gain1/1 -> "Nx "/1
